simulink model "DriveSource"  (R2020a)
settings: Solver=VariableStepAuto  StartTime=0.0  StopTime=10.0  RelTol=1e-3
undefined symbols (not defined in the file): Right
libraries: vehdynlibscenariocommon x5, simulink x1
settings Model: Creator=Administrator  LastModifiedBy=Administrator

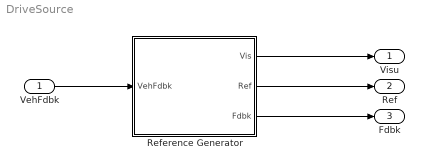
== system DriveSource ==
  VehFdbk : Inport  OutDataTypeStr=Bus: VehFdbk
  Reference Generator : Subsystem  Variant=on  VariantControlMode=Label  VariantControl=Variant1  LabelModeActiveChoice=4
  Visu : Outport
  Ref : Outport  Port=2
  Fdbk : Outport  Port=3
  wires:
  VehFdbk/1 -> Reference Generator/1("VehFdbk ")
  Reference Generator/1(" Vis") -> Visu/1
  Reference Generator/2(" Ref") -> Ref/1
  Reference Generator/3(" Fdbk") -> Fdbk/1

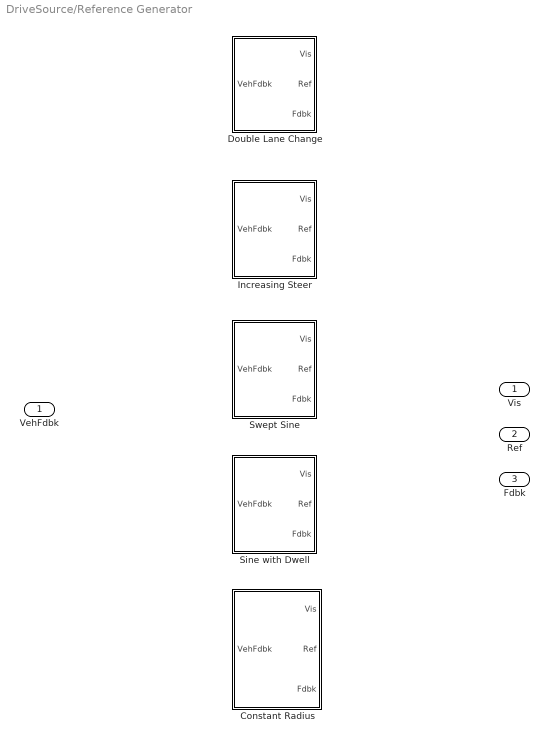
== system DriveSource/Reference Generator ==
  "VehFdbk " : Inport  OutDataTypeStr=Bus: VehFdbk
  Constant Radius : Subsystem  AncestorBlock=vehdynlibscenariocommon/Constant Radius  VariantControl=4  mask{t_start=0, xdot_r=120, xdotUnit=mph, R=22.5, turnDirMask=Right, ay_max=0.5, ay_stop=off, Parameter6=2}
      mask prompts: t_start "Maneuver start time, t_start [s]:"; xdot_r "Longitudinal velocity reference, xdot_r:"; xdotUnit "Longitudinal velocity reference units, xdotUnit []:"; R "Radius value, R [m]:"; turnDirMask "Turn direction"; ay_max "Lateral acceleration absolute threshold, ay_max [g]:"; ay_stop "Stop simulation at lateral acceleration threshold"
      mask TypeOptions xdotUnit: Longitudinal Velocity Reference/Input Units/Unit
      mask TypeOptions R: Constant Radius/Value
      mask TypeOptions turnDirMask: Constant Radius/turnDirMask
  Double Lane Change : Subsystem  VariantControl=0
  Increasing Steer : Subsystem  VariantControl=1
  Sine with Dwell : Subsystem  VariantControl=3
  Swept Sine : Subsystem  VariantControl=2
  " Vis" : Outport  VectorParamsAs1DForOutWhenUnconnected=off
  " Ref" : Outport  Port=2  VectorParamsAs1DForOutWhenUnconnected=off
  " Fdbk" : Outport  Port=3  VectorParamsAs1DForOutWhenUnconnected=off

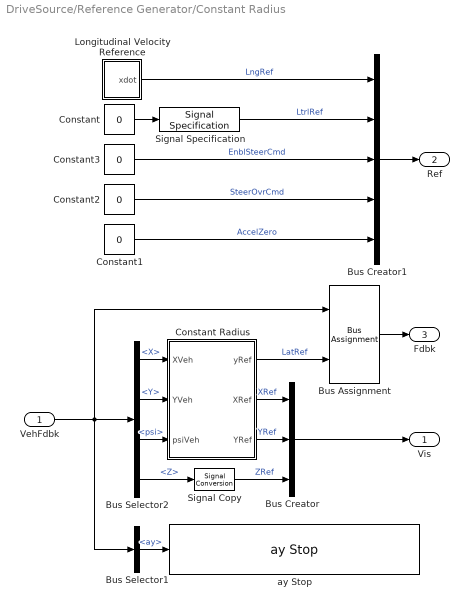
== system DriveSource/Reference Generator/Constant Radius ==
  "VehFdbk " : Inport  OutDataTypeStr=Bus: VehFdbk
  Bus Assignment : BusAssignment  AssignedSignals=Body.Y
  Bus Creator : BusCreator  Inputs=3
  Bus Creator1 : BusCreator  Inputs=5
  Bus Selector1 : BusSelector  OutputSignals=ay
  Bus Selector2 : BusSelector  OutputSignals=X,Y,psi,Z
  Constant : Constant  Value=0
  Constant Radius : Subsystem  mask{Value=R, turnDirMask=Right}
      mask prompts: Value "Simulink:blkprm_prompts:ConstConstValue"; turnDirMask "Turn direction"
      mask TypeOptions Value: R/Value
      mask TypeOptions turnDirMask: Left | Right
      mask DialogControl Value Prompt: Constant value:
  Constant1 : Constant  Value=0  OutDataTypeStr=boolean
  Constant2 : Constant  Value=0
  Constant3 : Constant  Value=0  OutDataTypeStr=boolean
  Longitudinal Velocity Reference : Subsystem
  Signal Copy : SignalConversion  OverrideOpt=off
  Signal Specification : SignalSpecification  Unit=m
  ay Stop : vehdynlibscenariocommon/Slowly Increasing Steer/ay Stop  SystemSampleTime=-1  Latency=0  AutoFrameSizeCalculation=off
      settings: SourceProductBaseCode=VE
  " Vis" : Outport  VectorParamsAs1DForOutWhenUnconnected=off
  " Ref" : Outport  Port=2  VectorParamsAs1DForOutWhenUnconnected=off
  " Fdbk" : Outport  Port=3  VectorParamsAs1DForOutWhenUnconnected=off
  wires:
  Constant3/1 -> Bus Creator1/3  "EnblSteerCmd"
  Constant2/1 -> Bus Creator1/4  "SteerOvrCmd"
  Longitudinal Velocity Reference/1(xdot) -> Bus Creator1/1  "LngRef"
  Signal Specification/1 -> Bus Creator1/2  "LtrlRef"
  Bus Creator1/1 -> " Ref"/1
  Constant1/1 -> Bus Creator1/5  "AccelZero"
  Constant/1 -> Signal Specification/1
  Constant Radius/1(yRef) -> Bus Assignment/2  "LatRef"
  Bus Assignment/1 -> " Fdbk"/1
  Signal Copy/1 -> Bus Creator/3  "ZRef"
  Bus Creator/1 -> " Vis"/1
  Bus Selector2/4 -> Signal Copy/1  "<Z>"
  Constant Radius/3(YRef) -> Bus Creator/2  "YRef"
  "VehFdbk "/1 -> Bus Selector2/1, Bus Assignment/1, Bus Selector1/1
  Bus Selector2/2 -> Constant Radius/2(YVeh)  "<Y>"
  Bus Selector2/3 -> Constant Radius/3(psiVeh)  "<psi>"
  Bus Selector2/1 -> Constant Radius/1(XVeh)  "<X>"
  Constant Radius/2(XRef) -> Bus Creator/1  "XRef"
  Bus Selector1/1 -> ay Stop/1  "<ay>"

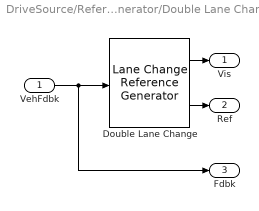
== system DriveSource/Reference Generator/Double Lane Change ==
  "VehFdbk " : Inport
  Double Lane Change : vehdynlibscenariocommon/Lane Change Reference Generator  VariantControl=Variant1  t_start=t_start  XGate=XGate  xdot_r=xdot_r  xdotUnit=mph  xStart=xStart  vehW=vehW  lattoff=lattoff  centerSwitch=on  latRefbp=latRefbp  latRef=latRef  aMode=2
      settings: SourceProductBaseCode=VE
  " Vis" : Outport  VectorParamsAs1DForOutWhenUnconnected=off
  " Ref" : Outport  Port=2  VectorParamsAs1DForOutWhenUnconnected=off
  " Fdbk" : Outport  Port=3  VectorParamsAs1DForOutWhenUnconnected=off
  wires:
  Double Lane Change/2 -> " Ref"/1
  Double Lane Change/1 -> " Vis"/1
  "VehFdbk "/1 -> Double Lane Change/1, " Fdbk"/1

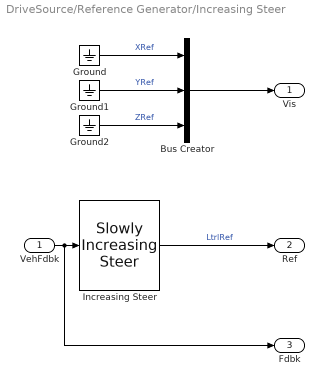
== system DriveSource/Reference Generator/Increasing Steer ==
  "VehFdbk " : Inport
  Bus Creator : BusCreator  Inputs=3
  Ground : Ground
  Ground1 : Ground
  Ground2 : Ground
  Increasing Steer : vehdynlibscenariocommon/Slowly Increasing Steer  VariantControl=1  t_start=t_start  xdot_r=xdot_r  xdotUnit=mph  omega_hw=omega_hw  theta_max=theta_max  t_stop=t_stop  ay_max=ay_max  ay_stop=on  aMode=2
      settings: SourceProductBaseCode=VE
  " Vis" : Outport  VectorParamsAs1DForOutWhenUnconnected=off
  " Ref" : Outport  Port=2  VectorParamsAs1DForOutWhenUnconnected=off
  " Fdbk" : Outport  Port=3  VectorParamsAs1DForOutWhenUnconnected=off
  wires:
  Ground/1 -> Bus Creator/1  "XRef"
  Ground1/1 -> Bus Creator/2  "YRef"
  Ground2/1 -> Bus Creator/3  "ZRef"
  Increasing Steer/1 -> " Ref"/1  "LtrlRef"
  Bus Creator/1 -> " Vis"/1
  "VehFdbk "/1 -> Increasing Steer/1, " Fdbk"/1

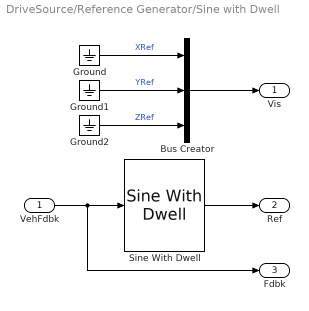
== system DriveSource/Reference Generator/Sine with Dwell ==
  "VehFdbk " : Inport
  Bus Creator : BusCreator  Inputs=3
  Ground : Ground
  Ground1 : Ground
  Ground2 : Ground
  Sine With Dwell : vehdynlibscenariocommon/Sine With Dwell  VariantControl=3  t_start=0  xdot_r=30  xdotUnit=mph  steerF=20  steerA=30  tdwell=5  steerDir=off  aMode=2
      settings: SourceProductBaseCode=VE
  " Vis" : Outport  VectorParamsAs1DForOutWhenUnconnected=off
  " Ref" : Outport  Port=2  VectorParamsAs1DForOutWhenUnconnected=off
  " Fdbk" : Outport  Port=3  VectorParamsAs1DForOutWhenUnconnected=off
  wires:
  Ground/1 -> Bus Creator/1  "XRef"
  Ground1/1 -> Bus Creator/2  "YRef"
  Ground2/1 -> Bus Creator/3  "ZRef"
  Bus Creator/1 -> " Vis"/1
  "VehFdbk "/1 -> Sine With Dwell/1, " Fdbk"/1
  Sine With Dwell/1 -> " Ref"/1

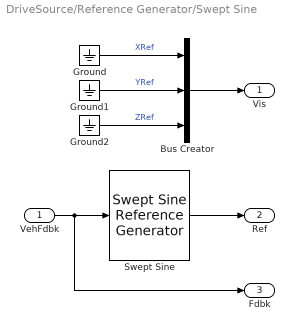
== system DriveSource/Reference Generator/Swept Sine ==
  "VehFdbk " : Inport
  Bus Creator : BusCreator  Inputs=3
  Ground : Ground
  Ground1 : Ground
  Ground2 : Ground
  Swept Sine : vehdynlibscenariocommon/Swept Sine Reference Generator  VariantControl=2  t_start=t_start  xdot_r=xdot_r  xdotUnit=mph  theta_hw=theta_hw  theta_hw_final=theta_hw_final  t_sweep=t_sweep  aMode=2
      settings: SourceProductBaseCode=VE
  " Vis" : Outport  VectorParamsAs1DForOutWhenUnconnected=off
  " Ref" : Outport  Port=2  VectorParamsAs1DForOutWhenUnconnected=off
  " Fdbk" : Outport  Port=3  VectorParamsAs1DForOutWhenUnconnected=off
  wires:
  Ground/1 -> Bus Creator/1  "XRef"
  Ground1/1 -> Bus Creator/2  "YRef"
  Ground2/1 -> Bus Creator/3  "ZRef"
  Bus Creator/1 -> " Vis"/1
  Swept Sine/1 -> " Ref"/1
  "VehFdbk "/1 -> Swept Sine/1, " Fdbk"/1

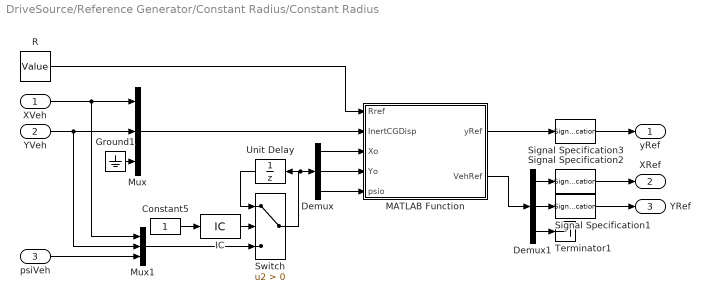
== system DriveSource/Reference Generator/Constant Radius/Constant Radius ==
  XVeh : Inport
  YVeh : Inport  Port=2
  psiVeh : Inport  Port=3
  Constant5 : Constant
  Demux : Demux  Outputs=3
  Demux1 : Demux  Outputs=3
  Ground1 : Ground
  IC : InitialCondition  Value=0
  MATLAB Function : MATLAB Function  TreatAsAtomicUnit=on
  Mux : Mux  Inputs=3
  Mux1 : Mux  Inputs=3
  R : Constant  Value=Value
  Signal Specification1 : SignalSpecification  Unit=m
  Signal Specification2 : SignalSpecification  Unit=m
  Signal Specification3 : SignalSpecification  Unit=m
  Switch : Switch  Criteria=u2 > Threshold
  Terminator1 : Terminator
  Unit Delay : UnitDelay  SampleTime=-1  HasFrameUpgradeWarning=on
  yRef : Outport  VectorParamsAs1DForOutWhenUnconnected=off
  XRef : Outport  Port=2  VectorParamsAs1DForOutWhenUnconnected=off
  YRef : Outport  Port=3  VectorParamsAs1DForOutWhenUnconnected=off
  wires:
  MATLAB Function/2(VehRef) -> Demux1/1
  Signal Specification3/1 -> yRef/1
  MATLAB Function/1(yRef) -> Signal Specification3/1
  Signal Specification2/1 -> XRef/1
  Signal Specification1/1 -> YRef/1
  Demux1/1 -> Signal Specification2/1
  Demux1/2 -> Signal Specification1/1
  Demux1/3 -> Terminator1/1
  psiVeh/1 -> Mux1/3
  R/1 -> MATLAB Function/1(Rref)
  Unit Delay/1 -> Switch/1
  Mux1/1 -> Switch/3
  IC/1 -> Switch/2
  Ground1/1 -> Mux/3
  Switch/1 -> Unit Delay/1, Demux/1
  Demux/1 -> MATLAB Function/3(Xo)
  Demux/3 -> MATLAB Function/5(psio)
  XVeh/1 -> Mux1/1, Mux/1
  Demux/2 -> MATLAB Function/4(Yo)
  YVeh/1 -> Mux1/2, Mux/2
  Constant5/1 -> IC/1
  Mux/1 -> MATLAB Function/2(InertCGDisp)

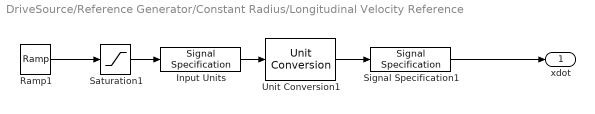
== system DriveSource/Reference Generator/Constant Radius/Longitudinal Velocity Reference ==
  Input Units : SignalSpecification  Unit=mph
  Ramp1 : simulink/Sources/Ramp  slope=100  start=t_start  InitialOutput=0
  Saturation1 : Saturate  UpperLimit=xdot_r  LowerLimit=0  ZeroCross=off
  Signal Specification1 : SignalSpecification  Unit=m/s
  Unit Conversion1 : UnitConversion
  xdot : Outport  VectorParamsAs1DForOutWhenUnconnected=off
  wires:
  Unit Conversion1/1 -> Signal Specification1/1
  Signal Specification1/1 -> xdot/1
  Saturation1/1 -> Input Units/1
  Ramp1/1 -> Saturation1/1
  Input Units/1 -> Unit Conversion1/1

== matlab function DriveSource/Reference Generator/Constant Radius/Constant Radius/MATLAB Function ==
  data: yRef output; Rref input; VehRef output size=3; InertCGDisp input; Xo input; Yo input; psio input; turnDirMask parameter
function [yRef,VehRef] = fcn(Rref, InertCGDisp,Xo,Yo,psio,turnDirMask)
if turnDirMask==1
    turnDir = 1;
else
    turnDir = -1;
end
Xo=Xo+Rref*sin(psio).*turnDir;
Yo=Yo-Rref*cos(psio).*turnDir;
RVeh = sqrt((InertCGDisp(1)-Xo).^2+(InertCGDisp(2)-Yo).^2);
theta = atan2(InertCGDisp(1)-Xo,InertCGDisp(2)-Yo)+atan2(0*2,RVeh).*turnDir;
VehRefX = Rref*sin(theta)+Xo;
VehRefY = Rref*cos(theta)+Yo;
VehRef = [VehRefX; VehRefY;InertCGDisp(3)];
yRef=-(Rref-RVeh).*turnDir;
% Rref = Rref.*turnDir;
% RVeh= RVeh.*turnDir;
